simulink model "MODEL_FULL_SYSTEM"  (Simulink 7.8)
settings: Solver=ode1  StartTime=0.0  StopTime=inf  FixedStep=Ts  MaxStep=1e-3  RelTol=1e-3
PostLoadFcn:
  | Ts=80e-6; relays_settings_init;
InitFcn:
  | Ts=80e-6; relays_settings_init;
values from neighbouring files (symbols this model uses):
  relay_sets = xlsread('relay_settings_10272015.xlsx')    [relays_settings_init.m]
undefined symbols (not defined in the file or in its folder): dfilt, DiscIntNeverNeededParam, fdesignblkfcn, gcbh, Left, opmodbus_cb, ph, Right, type, V, X
libraries: simulink x72, modbus_lib x40, cables_lib x36, rtio_opalrt_common x21, rtlab x20, transformer_lib x13, dynamic_load_lib x12, powerlib x6, simulink_extras x6, ssn_lib x5, discretizing x4, rteventslib x4
(part 2 of 7)

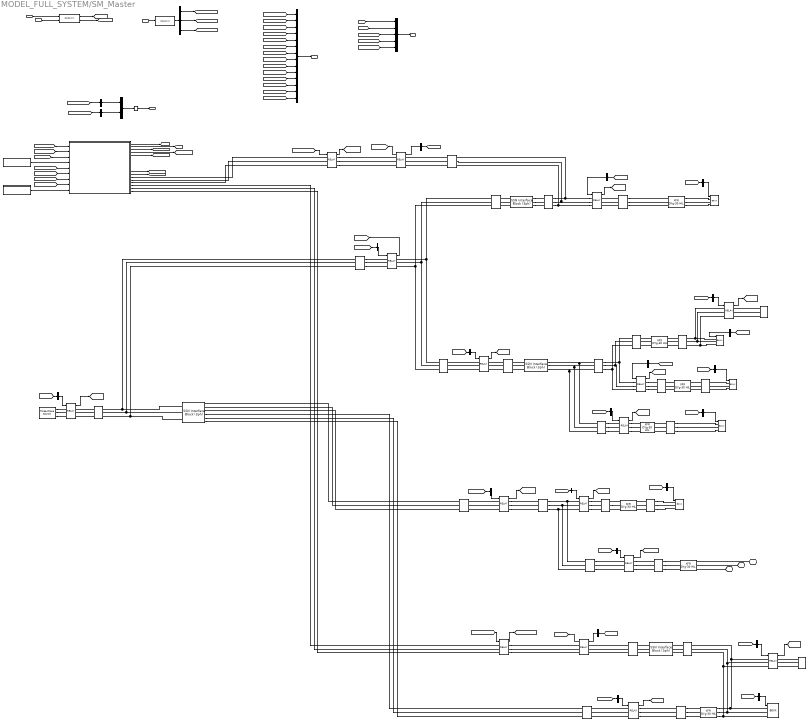
== system MODEL_FULL_SYSTEM/SM_Master ==
  SEL_787_IN : Inport
  LOAD_PQ_IN : Inport  Port=2
  IO ctrl : Inport  Port=3
  1/0AWG_L022 : cables_lib/1//0AWG_cable  length=1000  par_sets=1
  1/0AWG_cable1 : cables_lib/1//0AWG_cable  length=51  par_sets=1
  2/0AWG_L026L030 : cables_lib/2//0AWG_cable  length=1010  par_sets=1
  2000 kVA1 : transformer_lib/XFR DYg-30 HIL  Rating=2000  Vp=13800  Vs=460  Z=5.75  XR=5.7
  2000 kVA2 : transformer_lib/XFR DYg-30 HIL  Rating=2000  Vp=13800  Vs=460  Z=5.75  XR=5.7
  2000 kVA3 : transformer_lib/XFR DYg-30 HIL  Rating=2000  Vp=13800  Vs=460  Z=5.18  XR=2.5
  3750 kVA : transformer_lib/XFR DYg-30 HIL  Rating=3750  Vp=13800  Vs=4160  Z=4.75  XR=11.4
  3750 kVA3 : transformer_lib/XFR DYg-30 HIL  Rating=3750  Vp=13800  Vs=460  Z=4.75  XR=11.4
  4/0AWG_L027L028 : cables_lib/4//0AWG_cable  length=100  par_sets=1
  4/0AWG_L035L1 : cables_lib/4//0AWG_cable  length=1400  par_sets=1
  4/0AWG_L1 : cables_lib/4//0AWG_cable  length=25  par_sets=1
  4/0AWG_L2 : cables_lib/4//0AWG_cable  length=10  par_sets=1
  4/0AWG_L3 : cables_lib/4//0AWG_cable  length=150  par_sets=1
  500 kVA2 : transformer_lib/XFR DYg-30 HIL  Rating=500  Vp=13800  Vs=460  Z=5  XR=4.9
  500kcmil_L002 : cables_lib/500kcmil_cable  length=1851  par_sets=1
  500kcmil_L006 : cables_lib/500kcmil_cable  length=251  par_sets=1
  500kcmil_L018 : cables_lib/500kcmil_cable  length=1851  par_sets=1
  500kcmil_L1 : cables_lib/500kcmil_cable  length=125  par_sets=2
  500kcmil_L{2,7,10,14} (4 alike) : cables_lib/500kcmil_cable  length=50  par_sets=1
  500kcmil_L11 : cables_lib/500kcmil_cable  length=20  par_sets=1
  500kcmil_L12 : cables_lib/500kcmil_cable  length=10  par_sets=1
  500kcmil_L13 : cables_lib/500kcmil_cable  length=1  par_sets=1
  500kcmil_L3 : cables_lib/500kcmil_cable  length=100  par_sets=1
  500kcmil_L4 : cables_lib/500kcmil_cable  length=720  par_sets=1
  500kcmil_L5 : cables_lib/500kcmil_cable  length=350  par_sets=1
  500kcmil_L6 : cables_lib/500kcmil_cable  length=50  par_sets=2
  500kcmil_L8 : cables_lib/500kcmil_cable  length=1000  par_sets=1
  500kcmil_L9 : cables_lib/500kcmil_cable  length=51  par_sets=1
  750 kVA : transformer_lib/XFR DYg-30 HIL  Rating=750  Vp=13800  Vs=460  Z=5.57  XR=3.96
  B001 : dynamic_load_lib/B0XX  V=460  P_Scale=2  Q_Scale=2
  B004 : dynamic_load_lib/B0XX  V=460  P_Scale=2  Q_Scale=2
  B009 : dynamic_load_lib/B0XX  V=460  P_Scale=2  Q_Scale=2
  B010 : dynamic_load_lib/B0XX  V=460  P_Scale=1  Q_Scale=1
  B011 : dynamic_load_lib/B0XX  V=460  P_Scale=1  Q_Scale=1
  B022 : dynamic_load_lib/B0XX  V=460  P_Scale=1  Q_Scale=1
  Bus Creator1 : BusCreator  Inputs=14
  Bus Creator2 : BusCreator  Inputs=5
  Bus Creator3 : BusCreator  Inputs=2
  Bus Selector : BusSelector  OutputSignals=SEL_787_Relay1
  Bus Selector1 : BusSelector  OutputSignals=SEL_787_Relay3
  Bus Selector10 : BusSelector  OutputSignals=SEL_787_Relay18
  Bus Selector11 : BusSelector  OutputSignals=SEL_787_Relay7
  Bus Selector12 : BusSelector  OutputSignals=Woodward,test_controls,DOUT GR3
  Bus Selector13 : BusSelector  OutputSignals=gal_per_hr_1MVA
  Bus Selector14 : BusSelector  OutputSignals=gal_per_hr_4MVA
  Bus Selector15 : BusSelector  OutputSignals=SEL_787_Relay12
  Bus Selector16 : BusSelector  OutputSignals=PQ_B001
  Bus Selector17 : BusSelector  OutputSignals=SEL_787_Relay11
  Bus Selector2 : BusSelector  OutputSignals=SEL_787_Relay19
  Bus Selector20 : BusSelector  OutputSignals=PQ_B022
  Bus Selector21 : BusSelector  OutputSignals=PQ_B011
  Bus Selector22 : BusSelector  OutputSignals=PQ_B010
  Bus Selector23 : BusSelector  OutputSignals=PQ_B009
  Bus Selector27 : BusSelector  OutputSignals=PQ_B004
  Bus Selector3 : BusSelector  OutputSignals=SEL_787_Relay4
  Bus Selector4 : BusSelector  OutputSignals=SEL_787_Relay5
  Bus Selector5 : BusSelector  OutputSignals=SEL_787_Relay9
  Bus Selector6 : BusSelector  OutputSignals=SEL_787_Relay6
  Bus Selector7 : BusSelector  OutputSignals=SEL_787_Relay2
  Bus Selector8 : BusSelector  OutputSignals=SEL_787_Relay8
  Bus Selector9 : BusSelector  OutputSignals=SEL_787_Relay10
  GCB_1MVA : modbus_lib/RELAY  Ts=Ts
      link override Three-Phase V-I Measurement/Model/VI/Ia: GotoTag=LibraryTag_Ia
      link override Three-Phase V-I Measurement/Model/VI/Ib: GotoTag=LibraryTag_Ib
      link override Three-Phase V-I Measurement/Model/VI/Ic: GotoTag=LibraryTag_Ic
      link override Three-Phase V-I Measurement/Model/VI/Va: GotoTag=LibraryTag_Va
      link override Three-Phase V-I Measurement/Model/VI/Vb: GotoTag=LibraryTag_Vb
      link override Three-Phase V-I Measurement/Model/VI/Vc: GotoTag=LibraryTag_Vc
      link override Three-Phase V-I Measurement1/Model/VI/Ia: GotoTag=LibraryTag_Ia
      link override Three-Phase V-I Measurement1/Model/VI/Ib: GotoTag=LibraryTag_Ib
      link override Three-Phase V-I Measurement1/Model/VI/Ic: GotoTag=LibraryTag_Ic
      link override Three-Phase V-I Measurement1/Model/VI/Va: GotoTag=LibraryTag_Va
      link override Three-Phase V-I Measurement1/Model/VI/Vb: GotoTag=LibraryTag_Vb
      link override Three-Phase V-I Measurement1/Model/VI/Vc: GotoTag=LibraryTag_Vc
  GCB_4MVA : modbus_lib/RELAY  Ts=Ts
      link override Three-Phase V-I Measurement/Model/VI/Ia: GotoTag=LibraryTag_Ia
      link override Three-Phase V-I Measurement/Model/VI/Ib: GotoTag=LibraryTag_Ib
      link override Three-Phase V-I Measurement/Model/VI/Ic: GotoTag=LibraryTag_Ic
      link override Three-Phase V-I Measurement/Model/VI/Va: GotoTag=LibraryTag_Va
      link override Three-Phase V-I Measurement/Model/VI/Vb: GotoTag=LibraryTag_Vb
      link override Three-Phase V-I Measurement/Model/VI/Vc: GotoTag=LibraryTag_Vc
      link override Three-Phase V-I Measurement1/Model/VI/Ia: GotoTag=LibraryTag_Ia
      link override Three-Phase V-I Measurement1/Model/VI/Ib: GotoTag=LibraryTag_Ib
      link override Three-Phase V-I Measurement1/Model/VI/Ic: GotoTag=LibraryTag_Ic
      link override Three-Phase V-I Measurement1/Model/VI/Va: GotoTag=LibraryTag_Va
      link override Three-Phase V-I Measurement1/Model/VI/Vb: GotoTag=LibraryTag_Vb
      link override Three-Phase V-I Measurement1/Model/VI/Vc: GotoTag=LibraryTag_Vc
  GRID : powerlib/Electrical Sources/Three-Phase Source  Voltage=13970  PhaseAngle=0  Frequency=60  InternalConnection=Yg  SpecifyImpedance=on  Resistance=0.8929  Inductance=16.58e-3  ShortCircuitLevel=375e6  BaseVoltage=13800  XRratio=7.9  BusType=swing  Pref=0  Qref=0  Qmin=-inf  Qmax=inf
  Gen_initial_condition_1MVA : Subsystem
  Gen_initial_condition_4MVA : Subsystem
  Generator_09222015 : Subsystem
  Memory : Memory
  OpComm1 : rtlab/OpComm  nbport=2  groupe_acq=1  subsys_rate=0  st=0  Synchronization=on  Interpolation=on  Threshold=1.0  Missed_Data=off  Sim_Time=off  Samples=off  dynSigOut=off  from_console=0  warning_done=off  writeOpCommFile=off  Offset=off
  OpComm2 : rtlab/OpComm  nbport=1  groupe_acq=1  subsys_rate=0  st=0  Synchronization=on  Interpolation=on  Threshold=1.0  Missed_Data=off  Sim_Time=off  Samples=off  dynSigOut=off  from_console=1  warning_done=off  writeOpCommFile=off  Offset=off
  RELAY1 : modbus_lib/RELAY  Ts=Ts
      link override Three-Phase V-I Measurement/Model/VI/Ia: GotoTag=LibraryTag_Ia
      link override Three-Phase V-I Measurement/Model/VI/Ib: GotoTag=LibraryTag_Ib
      link override Three-Phase V-I Measurement/Model/VI/Ic: GotoTag=LibraryTag_Ic
      link override Three-Phase V-I Measurement/Model/VI/Va: GotoTag=LibraryTag_Va
      link override Three-Phase V-I Measurement/Model/VI/Vb: GotoTag=LibraryTag_Vb
      link override Three-Phase V-I Measurement/Model/VI/Vc: GotoTag=LibraryTag_Vc
      link override Three-Phase V-I Measurement1/Model/VI/Ia: GotoTag=LibraryTag_Ia
      link override Three-Phase V-I Measurement1/Model/VI/Ib: GotoTag=LibraryTag_Ib
      link override Three-Phase V-I Measurement1/Model/VI/Ic: GotoTag=LibraryTag_Ic
      link override Three-Phase V-I Measurement1/Model/VI/Va: GotoTag=LibraryTag_Va
      link override Three-Phase V-I Measurement1/Model/VI/Vb: GotoTag=LibraryTag_Vb
      link override Three-Phase V-I Measurement1/Model/VI/Vc: GotoTag=LibraryTag_Vc
  RELAY10 : modbus_lib/RELAY  Ts=Ts
      link override Three-Phase V-I Measurement/Model/VI/Ia: GotoTag=LibraryTag_Ia
      link override Three-Phase V-I Measurement/Model/VI/Ib: GotoTag=LibraryTag_Ib
      link override Three-Phase V-I Measurement/Model/VI/Ic: GotoTag=LibraryTag_Ic
      link override Three-Phase V-I Measurement/Model/VI/Va: GotoTag=LibraryTag_Va
      link override Three-Phase V-I Measurement/Model/VI/Vb: GotoTag=LibraryTag_Vb
      link override Three-Phase V-I Measurement/Model/VI/Vc: GotoTag=LibraryTag_Vc
      link override Three-Phase V-I Measurement1/Model/VI/Ia: GotoTag=LibraryTag_Ia
      link override Three-Phase V-I Measurement1/Model/VI/Ib: GotoTag=LibraryTag_Ib
      link override Three-Phase V-I Measurement1/Model/VI/Ic: GotoTag=LibraryTag_Ic
      link override Three-Phase V-I Measurement1/Model/VI/Va: GotoTag=LibraryTag_Va
      link override Three-Phase V-I Measurement1/Model/VI/Vb: GotoTag=LibraryTag_Vb
      link override Three-Phase V-I Measurement1/Model/VI/Vc: GotoTag=LibraryTag_Vc
  RELAY11 : modbus_lib/RELAY  Ts=Ts
      link override Three-Phase V-I Measurement/Model/VI/Ia: GotoTag=LibraryTag_Ia
      link override Three-Phase V-I Measurement/Model/VI/Ib: GotoTag=LibraryTag_Ib
      link override Three-Phase V-I Measurement/Model/VI/Ic: GotoTag=LibraryTag_Ic
      link override Three-Phase V-I Measurement/Model/VI/Va: GotoTag=LibraryTag_Va
      link override Three-Phase V-I Measurement/Model/VI/Vb: GotoTag=LibraryTag_Vb
      link override Three-Phase V-I Measurement/Model/VI/Vc: GotoTag=LibraryTag_Vc
      link override Three-Phase V-I Measurement1/Model/VI/Ia: GotoTag=LibraryTag_Ia
      link override Three-Phase V-I Measurement1/Model/VI/Ib: GotoTag=LibraryTag_Ib
      link override Three-Phase V-I Measurement1/Model/VI/Ic: GotoTag=LibraryTag_Ic
      link override Three-Phase V-I Measurement1/Model/VI/Va: GotoTag=LibraryTag_Va
      link override Three-Phase V-I Measurement1/Model/VI/Vb: GotoTag=LibraryTag_Vb
      link override Three-Phase V-I Measurement1/Model/VI/Vc: GotoTag=LibraryTag_Vc
  RELAY12 : modbus_lib/RELAY  Ts=Ts
      link override Three-Phase V-I Measurement/Model/VI/Ia: GotoTag=LibraryTag_Ia
      link override Three-Phase V-I Measurement/Model/VI/Ib: GotoTag=LibraryTag_Ib
      link override Three-Phase V-I Measurement/Model/VI/Ic: GotoTag=LibraryTag_Ic
      link override Three-Phase V-I Measurement/Model/VI/Va: GotoTag=LibraryTag_Va
      link override Three-Phase V-I Measurement/Model/VI/Vb: GotoTag=LibraryTag_Vb
      link override Three-Phase V-I Measurement/Model/VI/Vc: GotoTag=LibraryTag_Vc
      link override Three-Phase V-I Measurement1/Model/VI/Ia: GotoTag=LibraryTag_Ia
      link override Three-Phase V-I Measurement1/Model/VI/Ib: GotoTag=LibraryTag_Ib
      link override Three-Phase V-I Measurement1/Model/VI/Ic: GotoTag=LibraryTag_Ic
      link override Three-Phase V-I Measurement1/Model/VI/Va: GotoTag=LibraryTag_Va
      link override Three-Phase V-I Measurement1/Model/VI/Vb: GotoTag=LibraryTag_Vb
      link override Three-Phase V-I Measurement1/Model/VI/Vc: GotoTag=LibraryTag_Vc
  RELAY18 : modbus_lib/RELAY  Ts=Ts
      link override Three-Phase V-I Measurement/Model/VI/Ia: GotoTag=LibraryTag_Ia
      link override Three-Phase V-I Measurement/Model/VI/Ib: GotoTag=LibraryTag_Ib
      link override Three-Phase V-I Measurement/Model/VI/Ic: GotoTag=LibraryTag_Ic
      link override Three-Phase V-I Measurement/Model/VI/Va: GotoTag=LibraryTag_Va
      link override Three-Phase V-I Measurement/Model/VI/Vb: GotoTag=LibraryTag_Vb
      link override Three-Phase V-I Measurement/Model/VI/Vc: GotoTag=LibraryTag_Vc
      link override Three-Phase V-I Measurement1/Model/VI/Ia: GotoTag=LibraryTag_Ia
      link override Three-Phase V-I Measurement1/Model/VI/Ib: GotoTag=LibraryTag_Ib
      link override Three-Phase V-I Measurement1/Model/VI/Ic: GotoTag=LibraryTag_Ic
      link override Three-Phase V-I Measurement1/Model/VI/Va: GotoTag=LibraryTag_Va
      link override Three-Phase V-I Measurement1/Model/VI/Vb: GotoTag=LibraryTag_Vb
      link override Three-Phase V-I Measurement1/Model/VI/Vc: GotoTag=LibraryTag_Vc
  RELAY19 : modbus_lib/RELAY  Ts=Ts
      link override Three-Phase V-I Measurement/Model/VI/Ia: GotoTag=LibraryTag_Ia
      link override Three-Phase V-I Measurement/Model/VI/Ib: GotoTag=LibraryTag_Ib
      link override Three-Phase V-I Measurement/Model/VI/Ic: GotoTag=LibraryTag_Ic
      link override Three-Phase V-I Measurement/Model/VI/Va: GotoTag=LibraryTag_Va
      link override Three-Phase V-I Measurement/Model/VI/Vb: GotoTag=LibraryTag_Vb
      link override Three-Phase V-I Measurement/Model/VI/Vc: GotoTag=LibraryTag_Vc
      link override Three-Phase V-I Measurement1/Model/VI/Ia: GotoTag=LibraryTag_Ia
      link override Three-Phase V-I Measurement1/Model/VI/Ib: GotoTag=LibraryTag_Ib
      link override Three-Phase V-I Measurement1/Model/VI/Ic: GotoTag=LibraryTag_Ic
      link override Three-Phase V-I Measurement1/Model/VI/Va: GotoTag=LibraryTag_Va
      link override Three-Phase V-I Measurement1/Model/VI/Vb: GotoTag=LibraryTag_Vb
      link override Three-Phase V-I Measurement1/Model/VI/Vc: GotoTag=LibraryTag_Vc
  RELAY2 : modbus_lib/RELAY  Ts=Ts
      link override Three-Phase V-I Measurement/Model/VI/Ia: GotoTag=LibraryTag_Ia
      link override Three-Phase V-I Measurement/Model/VI/Ib: GotoTag=LibraryTag_Ib
      link override Three-Phase V-I Measurement/Model/VI/Ic: GotoTag=LibraryTag_Ic
      link override Three-Phase V-I Measurement/Model/VI/Va: GotoTag=LibraryTag_Va
      link override Three-Phase V-I Measurement/Model/VI/Vb: GotoTag=LibraryTag_Vb
      link override Three-Phase V-I Measurement/Model/VI/Vc: GotoTag=LibraryTag_Vc
      link override Three-Phase V-I Measurement1/Model/VI/Ia: GotoTag=LibraryTag_Ia
      link override Three-Phase V-I Measurement1/Model/VI/Ib: GotoTag=LibraryTag_Ib
      link override Three-Phase V-I Measurement1/Model/VI/Ic: GotoTag=LibraryTag_Ic
      link override Three-Phase V-I Measurement1/Model/VI/Va: GotoTag=LibraryTag_Va
      link override Three-Phase V-I Measurement1/Model/VI/Vb: GotoTag=LibraryTag_Vb
      link override Three-Phase V-I Measurement1/Model/VI/Vc: GotoTag=LibraryTag_Vc
  RELAY3 : modbus_lib/RELAY  Ts=Ts
      link override Three-Phase V-I Measurement/Model/VI/Ia: GotoTag=LibraryTag_Ia
      link override Three-Phase V-I Measurement/Model/VI/Ib: GotoTag=LibraryTag_Ib
      link override Three-Phase V-I Measurement/Model/VI/Ic: GotoTag=LibraryTag_Ic
      link override Three-Phase V-I Measurement/Model/VI/Va: GotoTag=LibraryTag_Va
      link override Three-Phase V-I Measurement/Model/VI/Vb: GotoTag=LibraryTag_Vb
      link override Three-Phase V-I Measurement/Model/VI/Vc: GotoTag=LibraryTag_Vc
      link override Three-Phase V-I Measurement1/Model/VI/Ia: GotoTag=LibraryTag_Ia
      link override Three-Phase V-I Measurement1/Model/VI/Ib: GotoTag=LibraryTag_Ib
      link override Three-Phase V-I Measurement1/Model/VI/Ic: GotoTag=LibraryTag_Ic
      link override Three-Phase V-I Measurement1/Model/VI/Va: GotoTag=LibraryTag_Va
      link override Three-Phase V-I Measurement1/Model/VI/Vb: GotoTag=LibraryTag_Vb
      link override Three-Phase V-I Measurement1/Model/VI/Vc: GotoTag=LibraryTag_Vc
  RELAY4 : modbus_lib/RELAY  Ts=Ts
      link override Three-Phase V-I Measurement/Model/VI/Ia: GotoTag=LibraryTag_Ia
      link override Three-Phase V-I Measurement/Model/VI/Ib: GotoTag=LibraryTag_Ib
      link override Three-Phase V-I Measurement/Model/VI/Ic: GotoTag=LibraryTag_Ic
      link override Three-Phase V-I Measurement/Model/VI/Va: GotoTag=LibraryTag_Va
      link override Three-Phase V-I Measurement/Model/VI/Vb: GotoTag=LibraryTag_Vb
      link override Three-Phase V-I Measurement/Model/VI/Vc: GotoTag=LibraryTag_Vc
      link override Three-Phase V-I Measurement1/Model/VI/Ia: GotoTag=LibraryTag_Ia
      link override Three-Phase V-I Measurement1/Model/VI/Ib: GotoTag=LibraryTag_Ib
      link override Three-Phase V-I Measurement1/Model/VI/Ic: GotoTag=LibraryTag_Ic
      link override Three-Phase V-I Measurement1/Model/VI/Va: GotoTag=LibraryTag_Va
      link override Three-Phase V-I Measurement1/Model/VI/Vb: GotoTag=LibraryTag_Vb
      link override Three-Phase V-I Measurement1/Model/VI/Vc: GotoTag=LibraryTag_Vc
  RELAY5 : modbus_lib/RELAY  Ts=Ts
      link override Three-Phase V-I Measurement/Model/VI/Ia: GotoTag=LibraryTag_Ia
      link override Three-Phase V-I Measurement/Model/VI/Ib: GotoTag=LibraryTag_Ib
      link override Three-Phase V-I Measurement/Model/VI/Ic: GotoTag=LibraryTag_Ic
      link override Three-Phase V-I Measurement/Model/VI/Va: GotoTag=LibraryTag_Va
      link override Three-Phase V-I Measurement/Model/VI/Vb: GotoTag=LibraryTag_Vb
      link override Three-Phase V-I Measurement/Model/VI/Vc: GotoTag=LibraryTag_Vc
      link override Three-Phase V-I Measurement1/Model/VI/Ia: GotoTag=LibraryTag_Ia
      link override Three-Phase V-I Measurement1/Model/VI/Ib: GotoTag=LibraryTag_Ib
      link override Three-Phase V-I Measurement1/Model/VI/Ic: GotoTag=LibraryTag_Ic
      link override Three-Phase V-I Measurement1/Model/VI/Va: GotoTag=LibraryTag_Va
      link override Three-Phase V-I Measurement1/Model/VI/Vb: GotoTag=LibraryTag_Vb
      link override Three-Phase V-I Measurement1/Model/VI/Vc: GotoTag=LibraryTag_Vc
  RELAY6 : modbus_lib/RELAY  Ts=Ts
      link override Three-Phase V-I Measurement/Model/VI/Ia: GotoTag=LibraryTag_Ia
      link override Three-Phase V-I Measurement/Model/VI/Ib: GotoTag=LibraryTag_Ib
      link override Three-Phase V-I Measurement/Model/VI/Ic: GotoTag=LibraryTag_Ic
      link override Three-Phase V-I Measurement/Model/VI/Va: GotoTag=LibraryTag_Va
      link override Three-Phase V-I Measurement/Model/VI/Vb: GotoTag=LibraryTag_Vb
      link override Three-Phase V-I Measurement/Model/VI/Vc: GotoTag=LibraryTag_Vc
      link override Three-Phase V-I Measurement1/Model/VI/Ia: GotoTag=LibraryTag_Ia
      link override Three-Phase V-I Measurement1/Model/VI/Ib: GotoTag=LibraryTag_Ib
      link override Three-Phase V-I Measurement1/Model/VI/Ic: GotoTag=LibraryTag_Ic
      link override Three-Phase V-I Measurement1/Model/VI/Va: GotoTag=LibraryTag_Va
      link override Three-Phase V-I Measurement1/Model/VI/Vb: GotoTag=LibraryTag_Vb
      link override Three-Phase V-I Measurement1/Model/VI/Vc: GotoTag=LibraryTag_Vc
  RELAY7 : modbus_lib/RELAY  Ts=Ts
      link override Three-Phase V-I Measurement/Model/VI/Ia: GotoTag=LibraryTag_Ia
      link override Three-Phase V-I Measurement/Model/VI/Ib: GotoTag=LibraryTag_Ib
      link override Three-Phase V-I Measurement/Model/VI/Ic: GotoTag=LibraryTag_Ic
      link override Three-Phase V-I Measurement/Model/VI/Va: GotoTag=LibraryTag_Va
      link override Three-Phase V-I Measurement/Model/VI/Vb: GotoTag=LibraryTag_Vb
      link override Three-Phase V-I Measurement/Model/VI/Vc: GotoTag=LibraryTag_Vc
      link override Three-Phase V-I Measurement1/Model/VI/Ia: GotoTag=LibraryTag_Ia
      link override Three-Phase V-I Measurement1/Model/VI/Ib: GotoTag=LibraryTag_Ib
      link override Three-Phase V-I Measurement1/Model/VI/Ic: GotoTag=LibraryTag_Ic
      link override Three-Phase V-I Measurement1/Model/VI/Va: GotoTag=LibraryTag_Va
      link override Three-Phase V-I Measurement1/Model/VI/Vb: GotoTag=LibraryTag_Vb
      link override Three-Phase V-I Measurement1/Model/VI/Vc: GotoTag=LibraryTag_Vc
  RELAY8 : modbus_lib/RELAY  Ts=Ts
      link override Three-Phase V-I Measurement/Model/VI/Ia: GotoTag=LibraryTag_Ia
      link override Three-Phase V-I Measurement/Model/VI/Ib: GotoTag=LibraryTag_Ib
      link override Three-Phase V-I Measurement/Model/VI/Ic: GotoTag=LibraryTag_Ic
      link override Three-Phase V-I Measurement/Model/VI/Va: GotoTag=LibraryTag_Va
      link override Three-Phase V-I Measurement/Model/VI/Vb: GotoTag=LibraryTag_Vb
      link override Three-Phase V-I Measurement/Model/VI/Vc: GotoTag=LibraryTag_Vc
      link override Three-Phase V-I Measurement1/Model/VI/Ia: GotoTag=LibraryTag_Ia
      link override Three-Phase V-I Measurement1/Model/VI/Ib: GotoTag=LibraryTag_Ib
      link override Three-Phase V-I Measurement1/Model/VI/Ic: GotoTag=LibraryTag_Ic
      link override Three-Phase V-I Measurement1/Model/VI/Va: GotoTag=LibraryTag_Va
      link override Three-Phase V-I Measurement1/Model/VI/Vb: GotoTag=LibraryTag_Vb
      link override Three-Phase V-I Measurement1/Model/VI/Vc: GotoTag=LibraryTag_Vc
  RELAY9 : modbus_lib/RELAY  Ts=Ts
      link override Three-Phase V-I Measurement/Model/VI/Ia: GotoTag=LibraryTag_Ia
      link override Three-Phase V-I Measurement/Model/VI/Ib: GotoTag=LibraryTag_Ib
      link override Three-Phase V-I Measurement/Model/VI/Ic: GotoTag=LibraryTag_Ic
      link override Three-Phase V-I Measurement/Model/VI/Va: GotoTag=LibraryTag_Va
      link override Three-Phase V-I Measurement/Model/VI/Vb: GotoTag=LibraryTag_Vb
      link override Three-Phase V-I Measurement/Model/VI/Vc: GotoTag=LibraryTag_Vc
      link override Three-Phase V-I Measurement1/Model/VI/Ia: GotoTag=LibraryTag_Ia
      link override Three-Phase V-I Measurement1/Model/VI/Ib: GotoTag=LibraryTag_Ib
      link override Three-Phase V-I Measurement1/Model/VI/Ic: GotoTag=LibraryTag_Ic
      link override Three-Phase V-I Measurement1/Model/VI/Va: GotoTag=LibraryTag_Va
      link override Three-Phase V-I Measurement1/Model/VI/Vb: GotoTag=LibraryTag_Vb
      link override Three-Phase V-I Measurement1/Model/VI/Vc: GotoTag=LibraryTag_Vc
  SSN Interface Block (3ph)1 : ssn_lib/SSN Interface Block (3ph)  nb_phase=3  nb_port=2  p1_type=V-type(Left)  p2_type=V-type (Right)  p3_type=X-type(Right)  p4_type=V-type(Left)  p5_type=V-type(Left)  p6_type=V-type(Left)  p7_type=V-type(Left)  p8_type=V-type(Left)  p9_type=V-type(Left)  p10_type=V-type(Left)  p11_type=V-type(Left)  p12_type=V-type(Left)  p13_type=V-type(Left)  p14_type=V-type(Left)  p15_type=V-type(Left)  p16_type=V-type(Left)  I_port_shunt_resistance=1e9
  SSN Interface Block (3ph)2 : ssn_lib/SSN Interface Block (3ph)  nb_phase=3  nb_port=2  p1_type=V-type(Left)  p2_type=V-type (Right)  p3_type=X-type(Right)  p4_type=V-type(Left)  p5_type=V-type(Left)  p6_type=V-type(Left)  p7_type=V-type(Left)  p8_type=V-type(Left)  p9_type=V-type(Left)  p10_type=V-type(Left)  p11_type=V-type(Left)  p12_type=V-type(Left)  p13_type=V-type(Left)  p14_type=V-type(Left)  p15_type=V-type(Left)  p16_type=V-type(Left)  I_port_shunt_resistance=1e9
  SSN Interface Block (3ph)3 : ssn_lib/SSN Interface Block (3ph)  nb_phase=3  nb_port=2  p1_type=V-type(Left)  p2_type=V-type (Right)  p3_type=X-type(Right)  p4_type=V-type(Left)  p5_type=V-type(Left)  p6_type=V-type(Left)  p7_type=V-type(Left)  p8_type=V-type(Left)  p9_type=V-type(Left)  p10_type=V-type(Left)  p11_type=V-type(Left)  p12_type=V-type(Left)  p13_type=V-type(Left)  p14_type=V-type(Left)  p15_type=V-type(Left)  p16_type=V-type(Left)  I_port_shunt_resistance=1e9
  SSN Interface Block (3ph)5 : ssn_lib/SSN Interface Block (3ph)  nb_phase=3  nb_port=3  p1_type=V-type(Left)  p2_type=V-type (Right)  p3_type=V-type (Right)  p4_type=V-type(Left)  p5_type=V-type(Left)  p6_type=V-type(Left)  p7_type=V-type(Left)  p8_type=V-type(Left)  p9_type=V-type(Left)  p10_type=V-type(Left)  p11_type=V-type(Left)  p12_type=V-type(Left)  p13_type=V-type(Left)  p14_type=V-type(Left)  p15_type=V-type(Left)  p16_type=V-type(Left)  I_port_shunt_resistance=1e9
  temp_1 : dynamic_load_lib/B0XX_constant  v=460  kVA=100  pf=0.90
  temp_2 : dynamic_load_lib/B0XX_constant  v=460  kVA=100  pf=0.90
  A : PMIOPort  Tag=PMCPort  Port=1  Side=Left
  B : PMIOPort  Tag=PMCPort  Port=2  Side=Left
  C : PMIOPort  Tag=PMCPort  Port=3  Side=Left
  MODBUS_OUT : Outport
  From Woodward : Outport  Port=2
  gen_fuel : Outport  Port=3
  wires:
  RELAY4/1 -> [MODBUS_4]
  RELAY9/1 -> [MODBUS_9]
  Bus Creator1/1 -> MODBUS_OUT/1
  SEL_787_IN/1 -> OpComm1/1
  RELAY1/1 -> [MODBUS_1]
  RELAY6/1 -> [MODBUS_6]
  RELAY5/1 -> [MODBUS_5]
  RELAY10/1 -> [MODBUS_10]
  [RELAY_IN] -> Bus Selector/1
  Bus Selector/1 -> RELAY1/1  "<SEL_787_Relay1>"
  [RELAY_IN] -> Bus Selector3/1
  Bus Selector3/1 -> RELAY4/1  "<SEL_787_Relay4>"
  [RELAY_IN] -> Bus Selector5/1
  Bus Selector5/1 -> RELAY9/1  "<SEL_787_Relay9>"
  [RELAY_IN] -> Bus Selector6/1
  Bus Selector6/1 -> RELAY6/1  "<SEL_787_Relay6>"
  [RELAY_IN] -> Bus Selector7/1
  Bus Selector7/1 -> RELAY2/1  "<SEL_787_Relay2>"
  [RELAY_IN] -> Bus Selector4/1
  Bus Selector4/1 -> RELAY5/1  "<SEL_787_Relay5>"
  [RELAY_IN] -> Bus Selector9/1
  Bus Selector9/1 -> RELAY10/1  "<SEL_787_Relay10>"
  RELAY2/1 -> [MODBUS_2]
  RELAY18/1 -> [MODBUS_18]
  OpComm1/1 -> [RELAY_IN]
  LOAD_PQ_IN/1 -> OpComm1/2
  OpComm1/2 -> [PQ_BUS_IN]
  [PQ_BUS_IN] -> Bus Selector20/1
  Bus Selector20/1 -> B022/1  "<PQ_B022>"
  [PQ_BUS_IN] -> Bus Selector21/1
  Bus Selector21/1 -> B011/1  "<PQ_B011>"
  [PQ_BUS_IN] -> Bus Selector22/1
  Bus Selector22/1 -> B010/1  "<PQ_B010>"
  [PQ_BUS_IN] -> Bus Selector23/1
  Bus Selector23/1 -> B009/1  "<PQ_B009>"
  Bus Selector1/1 -> RELAY3/1  "<SEL_787_Relay3>"
  [RELAY_IN] -> Bus Selector1/1
  RELAY3/1 -> [MODBUS_3]
  [RELAY_IN] -> Bus Selector2/1
  [RELAY_IN] -> Bus Selector10/1
  Bus Selector10/1 -> RELAY18/1  "<SEL_787_Relay18>"
  RELAY8/1 -> [MODBUS_8]
  RELAY7/1 -> [MODBUS_7]
  OpComm2/1 -> Bus Selector12/1
  Bus Selector12/1 -> [woodward]  "<Woodward>"
  IO ctrl/1 -> OpComm2/1
  Bus Selector12/3 -> [Dout_GR3]  "<DOUT GR3>"
  Bus Selector12/2 -> [brkcont]  "<test_controls>"
  [Ctrl] -> Bus Creator2/1  "Ctrl"
  [HWIds] -> Bus Creator2/2  "HWIds"
  [Gen1_pri_meas] -> Bus Creator2/3  "Gen1_primary"
  [Gen2_pri_meas] -> Bus Creator2/4  "Gen2_primary"
  [DIn_CH00_31] -> Bus Creator2/5  "Digital In"
  Bus Creator2/1 -> From Woodward/1
  Memory/1 -> gen_fuel/1  "gen_consumption"
  [RELAY_IN] -> Bus Selector8/1
  Bus Selector8/1 -> RELAY8/1  "<SEL_787_Relay8>"
  [RELAY_IN] -> Bus Selector11/1
  Bus Selector11/1 -> RELAY7/1  "<SEL_787_Relay7>"
  [Dout_GR3] -> Generator_09222015/1(Digital Outputs)
  [brkcont] -> Generator_09222015/2(Console Breakers)
  [woodward] -> Generator_09222015/3(Woodward Enable)
  Gen_initial_condition_4MVA/1(S) -> Generator_09222015/9(Manual Control Gen2 (opt))
  Gen_initial_condition_1MVA/1(S) -> Generator_09222015/4(Manual Control Gen1 (opt))
  [MODBUS_7] -> Generator_09222015/6(MCB1 V and I)
  [GCB_1MVA_MS] -> Generator_09222015/5(GCB1 V and I)
  [GCB_4MVA_MS] -> Generator_09222015/7(GCB2 V and I)
  [MODBUS_1] -> Generator_09222015/8(MCB2 V and I)
  Generator_09222015/3(Digital Inputs) -> [DIn_CH00_31]
  Generator_09222015/1(Error (opt)) -> [Ctrl]
  Generator_09222015/2(ID (opt)) -> [HWIds]
  Generator_09222015/4(Gen1 Monitor) -> [Gen1_pri_meas]
  Generator_09222015/5(Gen1 GCB Control) -> [Gen1_GCB_ctrl]
  Generator_09222015/11(Gen2 Monitor) -> [Gen2_pri_meas]
  Generator_09222015/12(Gen2 GCB Control) -> [Gen2_GCB_ctrl]
  [Gen1_pri_meas] -> Bus Selector13/1  "1MVA"
  [Gen2_pri_meas] -> Bus Selector14/1  "4MVA"
  Bus Selector13/1 -> Bus Creator3/1  "<gal_per_hr_1MVA>"
  Bus Selector14/1 -> Bus Creator3/2  "<gal_per_hr_4MVA>"
  Bus Creator3/1 -> Memory/1
  GCB_4MVA/1 -> [GCB_4MVA_MS]
  [Gen1_GCB_ctrl] -> GCB_1MVA/1
  GCB_1MVA/1 -> [GCB_1MVA_MS]
  [Gen2_GCB_ctrl] -> GCB_4MVA/1
  Bus Selector27/1 -> B004/1  "<PQ_B004>"
  [PQ_BUS_IN] -> Bus Selector27/1
  Bus Selector15/1 -> RELAY12/1  "<SEL_787_Relay12>"
  [RELAY_IN] -> Bus Selector15/1
  Bus Selector17/1 -> RELAY11/1  "<SEL_787_Relay11>"
  [RELAY_IN] -> Bus Selector17/1
  RELAY11/1 -> [MODBUS_11]
  RELAY12/1 -> [MODBUS_12]
  [MODBUS_1] -> Bus Creator1/1
  [MODBUS_2] -> Bus Creator1/2
  [MODBUS_3] -> Bus Creator1/3
  [MODBUS_4] -> Bus Creator1/4
  [MODBUS_5] -> Bus Creator1/5
  [MODBUS_6] -> Bus Creator1/6
  [MODBUS_7] -> Bus Creator1/7
  [MODBUS_8] -> Bus Creator1/8
  [MODBUS_9] -> Bus Creator1/9
  [MODBUS_10] -> Bus Creator1/10
  [MODBUS_11] -> Bus Creator1/11
  [MODBUS_12] -> Bus Creator1/12
  [MODBUS_18] -> Bus Creator1/13
  [MODBUS_19] -> Bus Creator1/14
  Bus Selector16/1 -> B001/1  "<PQ_B001>"
  [PQ_BUS_IN] -> Bus Selector16/1
  Bus Selector2/1 -> RELAY19/1  "<SEL_787_Relay19>"
  RELAY19/1 -> [MODBUS_19]
  connections:
  500kcmil_L006/LConn3 -- RELAY5/RConn3
  500kcmil_L006/LConn2 -- RELAY5/RConn2
  500kcmil_L006/LConn1 -- RELAY5/RConn1
  2000 kVA1/RConn1 -- B001/LConn1 -- 500kcmil_L10/RConn1 -- RELAY18/LConn1
  2000 kVA1/RConn2 -- B001/LConn2 -- 500kcmil_L10/RConn2 -- RELAY18/LConn2
  2000 kVA1/RConn3 -- B001/LConn3 -- 500kcmil_L10/RConn3 -- RELAY18/LConn3
  RELAY6/LConn1 -- 4/0AWG_L3/RConn1
  RELAY6/LConn2 -- 4/0AWG_L3/RConn2
  RELAY6/LConn3 -- 4/0AWG_L3/RConn3
  RELAY10/LConn2 -- 4/0AWG_L035L1/RConn2 -- 2/0AWG_L026L030/LConn2
  500kcmil_L6/LConn3 -- 500 kVA2/RConn3
  500kcmil_L6/LConn2 -- 500 kVA2/RConn2
  500kcmil_L6/LConn1 -- 500 kVA2/RConn1
  750 kVA/LConn1 -- 4/0AWG_L027L028/RConn1
  750 kVA/LConn2 -- 4/0AWG_L027L028/RConn2
  750 kVA/LConn3 -- 4/0AWG_L027L028/RConn3
  2000 kVA2/LConn1 -- 2/0AWG_L026L030/RConn1
  2000 kVA2/LConn2 -- 2/0AWG_L026L030/RConn2
  2000 kVA2/LConn3 -- 2/0AWG_L026L030/RConn3
  B010/LConn1 -- 500kcmil_L2/RConn1
  B010/LConn2 -- 500kcmil_L2/RConn2
  B010/LConn3 -- 500kcmil_L2/RConn3
  500kcmil_L2/LConn1 -- 750 kVA/RConn1
  500kcmil_L2/LConn2 -- 750 kVA/RConn2
  500kcmil_L2/LConn3 -- 750 kVA/RConn3
  500kcmil_L1/LConn3 -- 2000 kVA2/RConn3
  500kcmil_L1/LConn2 -- 2000 kVA2/RConn2
  500kcmil_L1/LConn1 -- 2000 kVA2/RConn1
  RELAY10/LConn3 -- 4/0AWG_L035L1/RConn3 -- 2/0AWG_L026L030/LConn3
  RELAY10/LConn1 -- 4/0AWG_L035L1/RConn1 -- 2/0AWG_L026L030/LConn1
  500kcmil_L8/RConn3 -- 2000 kVA1/LConn3
  500kcmil_L8/RConn2 -- 2000 kVA1/LConn2
  500kcmil_L8/RConn1 -- 2000 kVA1/LConn1
  RELAY4/LConn3 -- 500kcmil_L7/RConn3
  RELAY4/LConn2 -- 500kcmil_L7/RConn2
  RELAY4/LConn1 -- 500kcmil_L7/RConn1
  3750 kVA3/RConn3 -- B022/LConn3
  3750 kVA3/RConn2 -- B022/LConn2
  3750 kVA3/RConn1 -- B022/LConn1
  GRID/RConn3 -- RELAY1/LConn3
  GRID/RConn2 -- RELAY1/LConn2
  GRID/RConn1 -- RELAY1/LConn1
  RELAY10/RConn3 -- 4/0AWG_L027L028/LConn3
  RELAY10/RConn2 -- 4/0AWG_L027L028/LConn2
  RELAY10/RConn1 -- 4/0AWG_L027L028/LConn1
  RELAY4/RConn3 -- 500kcmil_L8/LConn3
  RELAY4/RConn2 -- 500kcmil_L8/LConn2
  RELAY4/RConn1 -- 500kcmil_L8/LConn1
  RELAY9/RConn3 -- 500 kVA2/LConn3
  RELAY9/RConn2 -- 500 kVA2/LConn2
  RELAY9/RConn1 -- 500 kVA2/LConn1
  4/0AWG_L1/RConn3 -- RELAY9/LConn3
  4/0AWG_L1/RConn2 -- RELAY9/LConn2
  4/0AWG_L1/RConn1 -- RELAY9/LConn1
  RELAY5/LConn3 -- 500kcmil_L11/RConn3 -- 500kcmil_L3/RConn3
  RELAY5/LConn2 -- 500kcmil_L11/RConn2 -- 500kcmil_L3/RConn2
  RELAY5/LConn1 -- 500kcmil_L11/RConn1 -- 500kcmil_L3/RConn1
  500kcmil_L6/RConn3 -- B009/LConn3
  500kcmil_L6/RConn2 -- B009/LConn2
  500kcmil_L6/RConn1 -- B009/LConn1
  4/0AWG_L3/LConn3 -- RELAY2/RConn3 -- 500kcmil_L13/LConn3
  4/0AWG_L3/LConn2 -- RELAY2/RConn2 -- 500kcmil_L13/LConn2
  4/0AWG_L3/LConn1 -- RELAY2/RConn1 -- 500kcmil_L13/LConn1
  4/0AWG_L1/LConn2 -- 4/0AWG_L035L1/LConn2 -- SSN Interface Block (3ph)1/RConn2
  SSN Interface Block (3ph)5/LConn3 -- 500kcmil_L5/RConn3 -- 500kcmil_L4/LConn3
  B011/LConn3 -- 500kcmil_L1/RConn3 -- RELAY19/LConn3
  B011/LConn2 -- 500kcmil_L1/RConn2 -- RELAY19/LConn2
  B011/LConn1 -- 500kcmil_L1/RConn1 -- RELAY19/LConn1
  500kcmil_L3/LConn3 -- RELAY8/LConn3
  500kcmil_L3/LConn2 -- RELAY8/LConn2
  500kcmil_L3/LConn1 -- RELAY8/LConn1
  500kcmil_L5/LConn3 -- RELAY1/RConn3
  500kcmil_L5/LConn2 -- RELAY1/RConn2
  500kcmil_L5/LConn1 -- RELAY1/RConn1
  RELAY3/LConn3 -- 500kcmil_L9/RConn3
  RELAY3/LConn2 -- 500kcmil_L9/RConn2
  RELAY3/LConn1 -- 500kcmil_L9/RConn1
  500kcmil_L006/RConn3 -- 3750 kVA3/LConn3
  500kcmil_L006/RConn2 -- 3750 kVA3/LConn2
  500kcmil_L006/RConn1 -- 3750 kVA3/LConn1
  GCB_4MVA/RConn3 -- RELAY8/RConn3
  GCB_4MVA/RConn2 -- RELAY8/RConn2
  GCB_4MVA/RConn1 -- RELAY8/RConn1
  GCB_1MVA/RConn3 -- RELAY7/RConn3
  GCB_1MVA/RConn2 -- RELAY7/RConn2
  GCB_1MVA/RConn1 -- RELAY7/RConn1
  4/0AWG_L1/LConn3 -- 4/0AWG_L035L1/LConn3 -- SSN Interface Block (3ph)1/RConn3
  4/0AWG_L1/LConn1 -- 4/0AWG_L035L1/LConn1 -- SSN Interface Block (3ph)1/RConn1
  4/0AWG_L2/LConn3 -- RELAY6/RConn3
  4/0AWG_L2/LConn2 -- RELAY6/RConn2
  4/0AWG_L2/LConn1 -- RELAY6/RConn1
  SSN Interface Block (3ph)1/LConn3 -- 4/0AWG_L2/RConn3
  SSN Interface Block (3ph)1/LConn2 -- 4/0AWG_L2/RConn2
  SSN Interface Block (3ph)1/LConn1 -- 4/0AWG_L2/RConn1
  SSN Interface Block (3ph)2/LConn3 -- 500kcmil_L13/RConn3
  SSN Interface Block (3ph)2/LConn2 -- 500kcmil_L13/RConn2
  SSN Interface Block (3ph)2/LConn1 -- 500kcmil_L13/RConn1
  SSN Interface Block (3ph)2/RConn3 -- 500kcmil_L11/LConn3
  SSN Interface Block (3ph)2/RConn2 -- 500kcmil_L11/LConn2
  SSN Interface Block (3ph)2/RConn1 -- 500kcmil_L11/LConn1
  SSN Interface Block (3ph)5/LConn2 -- 500kcmil_L5/RConn2 -- 500kcmil_L4/LConn2
  SSN Interface Block (3ph)5/LConn1 -- 500kcmil_L5/RConn1 -- 500kcmil_L4/LConn1
  500kcmil_L12/LConn3 -- RELAY7/LConn3
  500kcmil_L12/LConn2 -- RELAY7/LConn2
  500kcmil_L12/LConn1 -- RELAY7/LConn1
  SSN Interface Block (3ph)3/RConn3 -- 500kcmil_L12/RConn3
  SSN Interface Block (3ph)3/RConn2 -- 500kcmil_L12/RConn2
  SSN Interface Block (3ph)3/RConn1 -- 500kcmil_L12/RConn1
  500kcmil_L10/LConn3 -- SSN Interface Block (3ph)3/LConn3
  500kcmil_L10/LConn2 -- SSN Interface Block (3ph)3/LConn2
  500kcmil_L10/LConn1 -- SSN Interface Block (3ph)3/LConn1
  500kcmil_L4/RConn3 -- RELAY2/LConn3
  500kcmil_L4/RConn2 -- RELAY2/LConn2
  500kcmil_L4/RConn1 -- RELAY2/LConn1
  Generator_09222015/RConn6 -- GCB_1MVA/LConn3
  Generator_09222015/RConn5 -- GCB_1MVA/LConn2
  Generator_09222015/RConn4 -- GCB_1MVA/LConn1
  Generator_09222015/RConn3 -- GCB_4MVA/LConn3
  Generator_09222015/RConn2 -- GCB_4MVA/LConn2
  Generator_09222015/RConn1 -- GCB_4MVA/LConn1
  500kcmil_L002/RConn3 -- RELAY11/LConn3 -- 500kcmil_L14/LConn3
  500kcmil_L002/RConn2 -- RELAY11/LConn2 -- 500kcmil_L14/LConn2
  500kcmil_L002/RConn1 -- RELAY11/LConn1 -- 500kcmil_L14/LConn1
  1/0AWG_cable1/RConn1 -- B004/LConn1
  2000 kVA3/LConn3 -- 1/0AWG_L022/RConn3
  1/0AWG_cable1/RConn2 -- B004/LConn2
  500kcmil_L14/RConn1 -- RELAY12/LConn1
  RELAY12/RConn3 -- 500kcmil_L018/LConn3
  2000 kVA3/LConn1 -- 1/0AWG_L022/RConn1
  RELAY12/RConn1 -- 500kcmil_L018/LConn1
  RELAY12/RConn2 -- 500kcmil_L018/LConn2
  1/0AWG_cable1/LConn3 -- 2000 kVA3/RConn3
  1/0AWG_cable1/LConn2 -- 2000 kVA3/RConn2
  1/0AWG_cable1/LConn1 -- 2000 kVA3/RConn1
  1/0AWG_L022/RConn2 -- 2000 kVA3/LConn2
  RELAY11/RConn3 -- 1/0AWG_L022/LConn3
  RELAY11/RConn2 -- 1/0AWG_L022/LConn2
  RELAY11/RConn1 -- 1/0AWG_L022/LConn1
  500kcmil_L14/RConn3 -- RELAY12/LConn3
  RELAY12/LConn2 -- 500kcmil_L14/RConn2
  1/0AWG_cable1/RConn3 -- B004/LConn3
  500kcmil_L018/RConn3 -- 3750 kVA/LConn3
  500kcmil_L018/RConn2 -- 3750 kVA/LConn2
  500kcmil_L018/RConn1 -- 3750 kVA/LConn1
  RELAY3/RConn3 -- 500kcmil_L002/LConn3
  RELAY3/RConn2 -- 500kcmil_L002/LConn2
  RELAY3/RConn1 -- 500kcmil_L002/LConn1
  SSN Interface Block (3ph)5/RConn6 -- 500kcmil_L7/LConn3
  SSN Interface Block (3ph)5/RConn5 -- 500kcmil_L7/LConn2
  SSN Interface Block (3ph)5/RConn4 -- 500kcmil_L7/LConn1
  500kcmil_L9/LConn3 -- SSN Interface Block (3ph)5/RConn3
  500kcmil_L9/LConn2 -- SSN Interface Block (3ph)5/RConn2
  500kcmil_L9/LConn1 -- SSN Interface Block (3ph)5/RConn1
  A/RConn1 -- 3750 kVA/RConn1
  B/RConn1 -- 3750 kVA/RConn2
  C/RConn1 -- 3750 kVA/RConn3
  temp_2/LConn3 -- RELAY18/RConn3
  temp_2/LConn2 -- RELAY18/RConn2
  temp_2/LConn1 -- RELAY18/RConn1
  temp_1/LConn3 -- RELAY19/RConn3
  temp_1/LConn2 -- RELAY19/RConn2
  temp_1/LConn1 -- RELAY19/RConn1
